simulink model "new3"  (R2025a)
settings: Solver=VariableStepAuto  StartTime=0.0  StopTime=2  RelTol=1e-3
undefined symbols (not defined in the file): g, Rs, Rsl, Rw, Ry
libraries: fl_lib x40, nesl_utility x14, ee_lib x12, slpidlib x3, spsFirstOrderFilterLib x1, spsOnDelayLib x1, simulink x1, spsabctodq0Lib x1
settings Model: SimulationMode=accelerator  Creator=maska  LastModifiedBy=maska

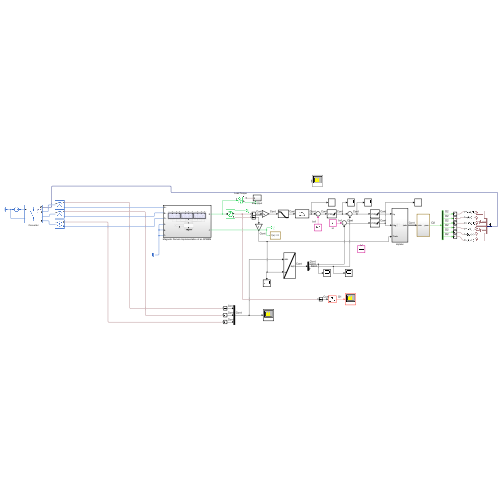
[thumbnail: Simulink's stored preview of the top-level diagram]
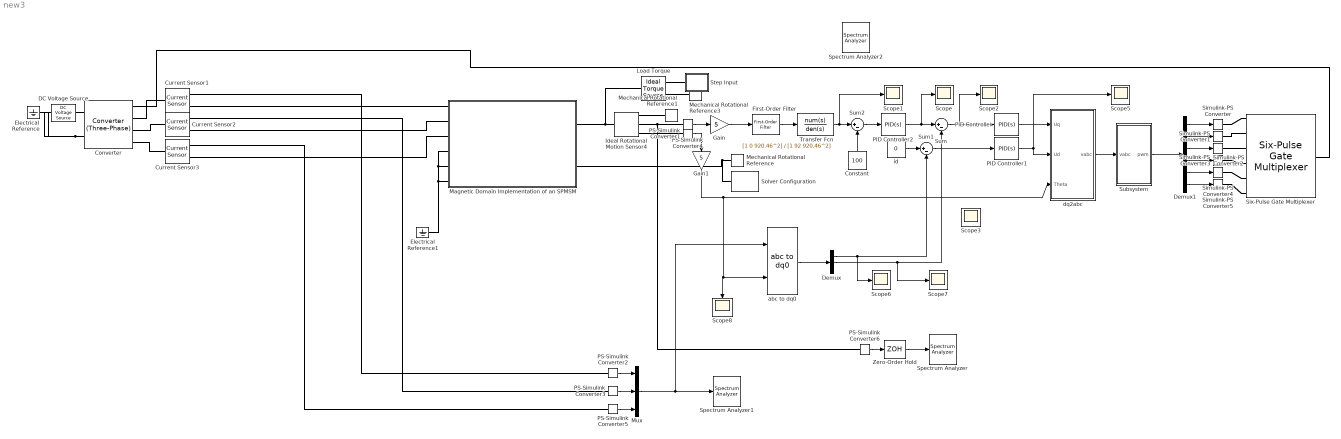
== system new3 ==
  Constant : Constant  Value=100
  Converter : ee_lib/Semiconductors & Converters/Converters/Converter (Three-Phase)  port_option=ee.enum.threePhasePort.expanded  fidelity_option=ee.enum.converters.fidelity.detailed  device_type=3  showThermalPort=false  K=0  Vth=0.5 V  Vgt=1 V  Vgt_off=-1 V  Ih=1 A  Vf=0.8 V  Ron=0.001 Ohm  Rds=0.001 Ohm  Goff=1e-5 1/Ohm  Eon_scalar=22.86e-3 J  Eoff_scalar=17.14e-3 J  Eoff_natural_commutation=10e-3 J  Voff=300 V  Iout_scalar=600 A  onCurrentMeasDelay=0 s  useCurrentFromPreviousCycle=false  useVoltageFromPreviousCycle=false  diode_param=2  diode_Vf=0.8 V  diode_Ron=0.001 Ohm  diode_Goff=1e-5 1/Ohm  diode_C=50 nF  diode_iRM=-235 A  diode_iF=300 A  diode_idot=-50 A/us  diode_trr_param=1  diode_trr_factor=3  diode_trr=15 us  diode_Qrr=1.5e+3 s*uA  diode_rec_loss_model=ee.enum.diode.reverseRecoveryModel.fixed  diode_ErecVal=0 J  diode_scaleWithIandV=false  diode_ErecMat=zeros(2, 3) J  diode_TjrecVec=[298.15, 398.15] K  diode_IfrecVec=[.1, 1, 10] A  diode_IrecVal=10 A  diode_VrecVal=10 V  diode_tFilter=1 / 1000 / 100 s  thermal_network_parameterization=ee.enum.thermalNetworkTopology.external  Rth=[.08, .5] K/W  Rth_Cauer=[.08, .1, .5] K/W  Rth_Foster=[.08, .14, .22, .16] K/W  thermal_mass_parameterization=ee.enum.thermalNetwork.timeconstant  thermal_mass=[.01, .5] J/K  thermal_mass_Cauer=[.01, .1, .5] J/K  thermal_mass_Foster=[.001, .005, .05, .5] J/K  thermal_time_constant=[.001, .2] s  thermal_time_constant_Cauer=[.001, .1, .2] s  thermal_time_constant_Foster=[7e-05, .0007, .01, .08] s  thermal_mass_initial_temperatures=[25, 25] degC  thermal_mass_initial_temperatures_Cauer=[25, 25, 25] degC  junction_thermal_mass=0.01 J/K  Tvec_initial_Foster=[25, 25, 25, 25] degC  snubber_type=0  Cs=1e-7 F  Rs=0.1 Ohm  Vce_loss=[0, 150, 300] V
      settings: InternalSimscapePortConfiguration="{\"Bottom\":[],\"Left\":[{\"id\":\"G\",\"label\":\"G\",\"type\":\"foundation.electrical.twelve_phase\"},{\"id\":\"a\",\"label\":\"a\",\"type\":\"foundation.electrical.electrical\"},{\"id\":\"b\",\"label\":\"b\",\"type\":\"foundation.electrical.electrical\"},{\"id\":\"c\",\"label\":\"c\",\"type\":\"foundation.electrical.electrical\"}],\"Right\":[{\"id\":\"p\",\"label\":\"+\",\"type\":\"foundation.electrical.electrical\"},{\"id\":\"n\",\"label\":\"-\",\"type\":\"foundation.electrical.electrical\"}],\"Top\":[]}"
  Current Sensor1 : fl_lib/Electrical/Electrical Sensors/Current Sensor
  Current Sensor2 : fl_lib/Electrical/Electrical Sensors/Current Sensor
  Current Sensor3 : fl_lib/Electrical/Electrical Sensors/Current Sensor
  DC Voltage Source : fl_lib/Electrical/Electrical Sources/DC Voltage Source  v0=750 V
  Demux : Demux  Outputs=3
  Demux1 : Demux  Outputs=6
  Electrical Reference : fl_lib/Electrical/Electrical Elements/Electrical Reference
  Electrical Reference1 : fl_lib/Electrical/Electrical Elements/Electrical Reference
  First-Order Filter : spsFirstOrderFilterLib/First-Order Filter  FilterType=Lowpass  Tc=0.04  Ts=0  Initialize=on  Vac_Init=[0, 0, 60]  Vdc_Init=0  PlotResponse=off  FreqRange="[0,  200,  1]"
  Gain : Gain  Gain=5
  Gain1 : Gain  Gain=5
  Ideal Rotational Motion Sensor4 : fl_lib/Mechanical/Mechanical Sensors/Ideal Rotational Motion Sensor  reference=foundation.enum.MeasurementReference.difference  acceleration_port=false  velocity_port=true  position_port=true  wrap_angle=false  offset=0 rad
  Load Torque : fl_lib/Mechanical/Mechanical Sources/Ideal Torque Source
  Magnetic Domain Implementation of an SPMSM : Subsystem
  Mechanical Rotational Reference : fl_lib/Mechanical/Rotational Elements/Mechanical Rotational Reference
  Mechanical Rotational Reference1 : fl_lib/Mechanical/Rotational Elements/Mechanical Rotational Reference
  Mechanical Rotational Reference3 : fl_lib/Mechanical/Rotational Elements/Mechanical Rotational Reference
  Mux : Mux  Inputs=3
  PID Controller : slpidlib/PID Controller  Controller=PID  Form=Parallel  TimeDomain=Continuous-time  UseExternalTs=off  SampleTime=-1  IntegratorMethod=Forward Euler  FilterMethod=Forward Euler  ControllerParametersSource=internal  P=1.95  I=0.85  UseKiTs=off  D=0  UseExternalDerivativeSource=off  N=100  UseFilter=on  TunerSelectOption=Transfer Function Based (PID Tuner App)  InitialConditionSource=internal  InitialConditionForIntegrator=0  InitialConditionForFilter=0  DifferentiatorICPrevScaledInput=0  ExternalReset=none  TrackingMode=off  Kt=1  LimitOutput=on  SatLimitsSource=internal  UpperSaturationLimit=1000  LowerSaturationLimit=-1000  LinearizeAsGain=on  AntiWindupMode=none  Kb=1  LimitIntegrator=on  UpperIntegratorSaturationLimit=100  LowerIntegratorSaturationLimit=-100  POutMin=[]  POutMax=[]  IOutMin=[]  IOutMax=[]  DOutMin=[]  DOutMax=[]  NOutMin=[]  NOutMax=[]  SumOutMin=[]  SumOutMax=[]  SaturationOutMin=[]  SaturationOutMax=[]  PParamMin=[]  PParamMax=[]  IParamMin=[]  IParamMax=[]  DParamMin=[]  DParamMax=[]  NParamMin=[]  NParamMax=[]  KbParamMin=[]  KbParamMax=[]  KtParamMin=[]  KtParamMax=[]  KbOutMin=[]  KbOutMax=[]  KtOutMin=[]  KtOutMax=[]  IntegratorOutMin=[]  IntegratorOutMax=[]  FilterOutMin=[]  FilterOutMax=[]  SumI1OutMin=[]  SumI1OutMax=[]  SumI2OutMin=[]  SumI2OutMax=[]  SumI3OutMin=[]  SumI3OutMax=[]  SumI4OutMin=[]  SumI4OutMax=[]  SumDOutMin=[]  SumDOutMax=[]  DifferentiatorOutMin=[]  DifferentiatorOutMax=[]  FilterDiffOutCoefMin=[]  FilterDiffOutCoefMax=[]  ReciprocalOutMin=[]  ReciprocalOutMax=[]  SumDenOutMin=[]  SumDenOutMax=[]  SumNumOutMin=[]  SumNumOutMax=[]  DivideOutMin=[]  DivideOutMax=[]  UdiffTsProdOutMin=[]  UdiffTsProdOutMax=[]  NTsProdOutMin=[]  NTsProdOutMax=[]  UintegralTsProdOutMin=[]  UintegralTsProdOutMax=[]  UngainTsProdOutMin=[]  UngainTsProdOutMax=[]  ClampingZeroOutDataTypeStr=Inherit: Inherit via back propagation  ClampingZeroOutMin=[]  ClampingZeroOutMax=[]  FilterDenConstantOutDataTypeStr=Inherit: Inherit via back propagation  FilterDenConstantOutMin=[]  FilterDenConstantOutMax=[]  PCopyOutDataTypeStr=Inherit: Inherit via back propagation  PCopyOutMin=[]  PCopyOutMax=[]  NCopyOutDataTypeStr=Inherit: Inherit via back propagation  NCopyOutMin=[]  NCopyOutMax=[]  IntegratorContinuousStateAttributes=''  IntegratorStateMustResolveToSignalObject=off  IntegratorRTWStateStorageClass=Auto  FilterContinuousStateAttributes=''  FilterStateMustResolveToSignalObject=off  FilterRTWStateStorageClass=Auto  ParallelPVariant=InternalParameters  IdealPVariant=Disabled  IVariant=InternalParameters  DVariant=InternalParameters  IntegratorVariant=Continuous  SatVariant=Enabled  AWVariant=Passthrough  PCopyVariant=Disabled  TRVariant=Disabled  FdbkBlocksVariant=Forward  IdealPFdbkVariant=Disabled  SatFdbkVariant=Disabled  DerivativeFilterVariant=ContFilter  NVariant=InternalParameters  NCopyVariant=Disabled  FilterICVariant=InternalICsFilter  IntegratorICVariant=InternalICs  ExternalResetVariant=Disabled  TRSumVariant=Passthrough  SumFdbkVariant=Disabled  SumVariant=Sum_PID  TsampFilterVariant=InternalTs  TsampNgainVariant=Passthrough  TsampIntegralVariant=Disabled_SignalSpec  ExternalSaturationOutDataTypeStr=Inherit: Same as second input  DerivativeSourceVariant=ErrorSignal  PreIntVariant=InternalPreInt
  PID Controller1 : slpidlib/PID Controller  Controller=PID  Form=Parallel  TimeDomain=Continuous-time  UseExternalTs=off  SampleTime=-1  IntegratorMethod=Forward Euler  FilterMethod=Forward Euler  ControllerParametersSource=internal  P=1.95  I=0.85  UseKiTs=off  D=0  UseExternalDerivativeSource=off  N=100  UseFilter=on  TunerSelectOption=Transfer Function Based (PID Tuner App)  InitialConditionSource=internal  InitialConditionForIntegrator=0  InitialConditionForFilter=0  DifferentiatorICPrevScaledInput=0  ExternalReset=none  TrackingMode=off  Kt=1  LimitOutput=on  SatLimitsSource=internal  UpperSaturationLimit=1000  LowerSaturationLimit=-1000  LinearizeAsGain=on  AntiWindupMode=none  Kb=1  LimitIntegrator=on  UpperIntegratorSaturationLimit=100  LowerIntegratorSaturationLimit=-100  POutMin=[]  POutMax=[]  IOutMin=[]  IOutMax=[]  DOutMin=[]  DOutMax=[]  NOutMin=[]  NOutMax=[]  SumOutMin=[]  SumOutMax=[]  SaturationOutMin=[]  SaturationOutMax=[]  PParamMin=[]  PParamMax=[]  IParamMin=[]  IParamMax=[]  DParamMin=[]  DParamMax=[]  NParamMin=[]  NParamMax=[]  KbParamMin=[]  KbParamMax=[]  KtParamMin=[]  KtParamMax=[]  KbOutMin=[]  KbOutMax=[]  KtOutMin=[]  KtOutMax=[]  IntegratorOutMin=[]  IntegratorOutMax=[]  FilterOutMin=[]  FilterOutMax=[]  SumI1OutMin=[]  SumI1OutMax=[]  SumI2OutMin=[]  SumI2OutMax=[]  SumI3OutMin=[]  SumI3OutMax=[]  SumI4OutMin=[]  SumI4OutMax=[]  SumDOutMin=[]  SumDOutMax=[]  DifferentiatorOutMin=[]  DifferentiatorOutMax=[]  FilterDiffOutCoefMin=[]  FilterDiffOutCoefMax=[]  ReciprocalOutMin=[]  ReciprocalOutMax=[]  SumDenOutMin=[]  SumDenOutMax=[]  SumNumOutMin=[]  SumNumOutMax=[]  DivideOutMin=[]  DivideOutMax=[]  UdiffTsProdOutMin=[]  UdiffTsProdOutMax=[]  NTsProdOutMin=[]  NTsProdOutMax=[]  UintegralTsProdOutMin=[]  UintegralTsProdOutMax=[]  UngainTsProdOutMin=[]  UngainTsProdOutMax=[]  ClampingZeroOutDataTypeStr=Inherit: Inherit via back propagation  ClampingZeroOutMin=[]  ClampingZeroOutMax=[]  FilterDenConstantOutDataTypeStr=Inherit: Inherit via back propagation  FilterDenConstantOutMin=[]  FilterDenConstantOutMax=[]  PCopyOutDataTypeStr=Inherit: Inherit via back propagation  PCopyOutMin=[]  PCopyOutMax=[]  NCopyOutDataTypeStr=Inherit: Inherit via back propagation  NCopyOutMin=[]  NCopyOutMax=[]  IntegratorContinuousStateAttributes=''  IntegratorStateMustResolveToSignalObject=off  IntegratorRTWStateStorageClass=Auto  FilterContinuousStateAttributes=''  FilterStateMustResolveToSignalObject=off  FilterRTWStateStorageClass=Auto  ParallelPVariant=InternalParameters  IdealPVariant=Disabled  IVariant=InternalParameters  DVariant=InternalParameters  IntegratorVariant=Continuous  SatVariant=Enabled  AWVariant=Passthrough  PCopyVariant=Disabled  TRVariant=Disabled  FdbkBlocksVariant=Forward  IdealPFdbkVariant=Disabled  SatFdbkVariant=Disabled  DerivativeFilterVariant=ContFilter  NVariant=InternalParameters  NCopyVariant=Disabled  FilterICVariant=InternalICsFilter  IntegratorICVariant=InternalICs  ExternalResetVariant=Disabled  TRSumVariant=Passthrough  SumFdbkVariant=Disabled  SumVariant=Sum_PID  TsampFilterVariant=InternalTs  TsampNgainVariant=Passthrough  TsampIntegralVariant=Disabled_SignalSpec  ExternalSaturationOutDataTypeStr=Inherit: Same as second input  DerivativeSourceVariant=ErrorSignal  PreIntVariant=InternalPreInt
  PID Controller2 : slpidlib/PID Controller  Controller=PID  Form=Parallel  TimeDomain=Continuous-time  UseExternalTs=off  SampleTime=-1  IntegratorMethod=Forward Euler  FilterMethod=Forward Euler  ControllerParametersSource=internal  P=0.008  I=0.00007  UseKiTs=off  D=0  UseExternalDerivativeSource=off  N=100  UseFilter=on  TunerSelectOption=Transfer Function Based (PID Tuner App)  InitialConditionSource=internal  InitialConditionForIntegrator=0  InitialConditionForFilter=0  DifferentiatorICPrevScaledInput=0  ExternalReset=none  TrackingMode=off  Kt=1  LimitOutput=on  SatLimitsSource=internal  UpperSaturationLimit=100  LowerSaturationLimit=-100  LinearizeAsGain=on  AntiWindupMode=none  Kb=1  LimitIntegrator=on  UpperIntegratorSaturationLimit=100  LowerIntegratorSaturationLimit=-100  POutMin=[]  POutMax=[]  IOutMin=[]  IOutMax=[]  DOutMin=[]  DOutMax=[]  NOutMin=[]  NOutMax=[]  SumOutMin=[]  SumOutMax=[]  SaturationOutMin=[]  SaturationOutMax=[]  PParamMin=[]  PParamMax=[]  IParamMin=[]  IParamMax=[]  DParamMin=[]  DParamMax=[]  NParamMin=[]  NParamMax=[]  KbParamMin=[]  KbParamMax=[]  KtParamMin=[]  KtParamMax=[]  KbOutMin=[]  KbOutMax=[]  KtOutMin=[]  KtOutMax=[]  IntegratorOutMin=[]  IntegratorOutMax=[]  FilterOutMin=[]  FilterOutMax=[]  SumI1OutMin=[]  SumI1OutMax=[]  SumI2OutMin=[]  SumI2OutMax=[]  SumI3OutMin=[]  SumI3OutMax=[]  SumI4OutMin=[]  SumI4OutMax=[]  SumDOutMin=[]  SumDOutMax=[]  DifferentiatorOutMin=[]  DifferentiatorOutMax=[]  FilterDiffOutCoefMin=[]  FilterDiffOutCoefMax=[]  ReciprocalOutMin=[]  ReciprocalOutMax=[]  SumDenOutMin=[]  SumDenOutMax=[]  SumNumOutMin=[]  SumNumOutMax=[]  DivideOutMin=[]  DivideOutMax=[]  UdiffTsProdOutMin=[]  UdiffTsProdOutMax=[]  NTsProdOutMin=[]  NTsProdOutMax=[]  UintegralTsProdOutMin=[]  UintegralTsProdOutMax=[]  UngainTsProdOutMin=[]  UngainTsProdOutMax=[]  ClampingZeroOutDataTypeStr=Inherit: Inherit via back propagation  ClampingZeroOutMin=[]  ClampingZeroOutMax=[]  FilterDenConstantOutDataTypeStr=Inherit: Inherit via back propagation  FilterDenConstantOutMin=[]  FilterDenConstantOutMax=[]  PCopyOutDataTypeStr=Inherit: Inherit via back propagation  PCopyOutMin=[]  PCopyOutMax=[]  NCopyOutDataTypeStr=Inherit: Inherit via back propagation  NCopyOutMin=[]  NCopyOutMax=[]  IntegratorContinuousStateAttributes=''  IntegratorStateMustResolveToSignalObject=off  IntegratorRTWStateStorageClass=Auto  FilterContinuousStateAttributes=''  FilterStateMustResolveToSignalObject=off  FilterRTWStateStorageClass=Auto  ParallelPVariant=InternalParameters  IdealPVariant=Disabled  IVariant=InternalParameters  DVariant=InternalParameters  IntegratorVariant=Continuous  SatVariant=Enabled  AWVariant=Passthrough  PCopyVariant=Disabled  TRVariant=Disabled  FdbkBlocksVariant=Forward  IdealPFdbkVariant=Disabled  SatFdbkVariant=Disabled  DerivativeFilterVariant=ContFilter  NVariant=InternalParameters  NCopyVariant=Disabled  FilterICVariant=InternalICsFilter  IntegratorICVariant=InternalICs  ExternalResetVariant=Disabled  TRSumVariant=Passthrough  SumFdbkVariant=Disabled  SumVariant=Sum_PID  TsampFilterVariant=InternalTs  TsampNgainVariant=Passthrough  TsampIntegralVariant=Disabled_SignalSpec  ExternalSaturationOutDataTypeStr=Inherit: Same as second input  DerivativeSourceVariant=ErrorSignal  PreIntVariant=InternalPreInt
  PS-Simulink Converter{1..6} (6 alike) : nesl_utility/PS-Simulink Converter  PhysicalDomain=network_engine_domain  SubClassName=ps_output  LeftPortType=input  RightPortType=output  PseudoPeriodic=off  Frequencies=[]  VectorFormat=inherit  Unit=inherit  AffineConversion=off
  Scope{,1..3,5..8} (8 alike) : Scope
      Scope settings: ActiveDisplayYMinimum=-4.019417563087452  ActiveDisplayYMaximum=1.1746832168582009
      Scope1 settings: ActiveDisplayYMinimum=-11.267228325018072  ActiveDisplayYMaximum=101.40505492516266
      Scope2 settings: ActiveDisplayYMinimum=-27.834658782595159  ActiveDisplayYMaximum=26.640626012143759  DataLoggingVariableName=ScopeData2
      Scope3 settings: ActiveDisplayYMinimum=-20.005283078213854  ActiveDisplayYMaximum=19.374157195669472  DataLoggingVariableName=ScopeData3
      Scope5 settings: ActiveDisplayYMinimum=-53.508802129582079  ActiveDisplayYMaximum=53.186558135240951  DataLoggingVariableName=ScopeData5
      Scope6 settings: ActiveDisplayYMinimum=-1437.9474938047751  ActiveDisplayYMaximum=1776.8392107438344  DataLoggingVariableName=ScopeData6
      Scope7 settings: ActiveDisplayYMinimum=-2.8426588150958878  ActiveDisplayYMaximum=1.0409285736394622  DataLoggingVariableName=ScopeData7
      Scope8 settings: ActiveDisplayYMinimum=10.636225564991161  ActiveDisplayYMaximum=10.664194284729955  DataLoggingVariableName=ScopeData8
  Simulink-PS Converter{,1..5} (6 alike) : nesl_utility/Simulink-PS Converter  PhysicalDomain=network_engine_domain  SubClassName=ps_input  LeftPortType=input  RightPortType=output  PseudoPeriodic=off  Frequencies=[]  NoiseDistribution=none  NoiseParameters=[]  Unit=1  AffineConversion=off  FilteringAndDerivatives=provide  SimscapeFilterOrder=1  InputFilterTimeConstant=0.001  UdotUserProvided=0
  Six-Pulse Gate Multiplexer : ee_lib/Semiconductors & Converters/Converters/Six-Pulse Gate Multiplexer  port_option=ee.enum.controlport.ps
  Solver Configuration : nesl_utility/Solver Configuration  PhysicalDomain=network_engine_domain  SubClassName=solver  LeftPortType=input  RightPortType=generic  Tones=[]  Harmonics=[]  SimulateNoise=off  Profile=off  UseLocalSampling=off  EnableSwitchedLinearOptims=on  FrequencyDomain=off  UseCCode=off  RelTol=0.001  AbsTol=1e-06  MinStep=1e-09  ToWorkspace=off  RevertToSquareIcSolve=off  NumHomotopyIterations=100  PhasorMode=off  PhasorModeNumHarmonics=1  ConsistencySolver=NEWTON_FTOL  IndexReductionMethod=DerivativeReplacement  DoDC=off  ResidualTolerance=1e-09  ConsistencyTolSource=GLOBAL  ConsistencyAbsTol=0.001  ConsistencyRelTol=0.001  ConsistencyTolFactor=0.001  UseLocalSolver=off  LocalSolverChoice=NE_BACKWARD_EULER_ADVANCER  ResolveIndetEquations=on  FunctionEvalNumThread=1  LocalSolverSampleTime=0.0001  DoFixedCost=off  MaxNonlinIter=3  MaxModeIter=2  ComputeImpulses=off  ImpulseIterations=1  LinearAlgebra=auto  LinearAlgebraNumThread=0  EquationFormulation=NE_TIME_EF  DelaysMemoryBudget=1024  AutomaticFiltering=on  FilteringTimeConstant=0.001  PartitionStorageMethod=AS_NEEDED  PartitionMemoryBudget=1024  PartitionMethod=ROBUST  MultibodyUseLocalSolver=off  MultibodyLocalSolverChoice=ODE1  MultibodyLocalSolverSampleTime=0.001
  Spectrum Analyzer : SpectrumAnalyzer  WindowPosition=[231.000000,114.000000,800.000000,483.000000,]  ScopeFrameLocation=window  SampleRate=44.1e3  PlotAsTwoSidedSpectrum=off  FrequencyScale=Log  WindowInvariantSamplesPerUpdate=on  FrequencySpan=Start and stop frequencies  StartFrequency=0  StopFrequency=50000  MaximizeAxes=Off  YLimits=[-34.3366 63.0554]  SelectedToolstripTab=spectrumAnalyzerToolstrip.measurementsTab
  Spectrum Analyzer1 : SpectrumAnalyzer  WindowPosition=[37.000000,290.000000,800.000000,483.000000,]  ScopeFrameLocation=window  SampleRate=44.1e3  PlotAsTwoSidedSpectrum=off  FrequencyScale=Log  WindowInvariantSamplesPerUpdate=on  FrequencySpan=Start and stop frequencies  StartFrequency=0  StopFrequency=50000  MaximizeAxes=Off  YLimits=[-64.8278 131.059]  SelectedToolstripTab=spectrumAnalyzerToolstrip.measurementsTab
  Spectrum Analyzer2 : SpectrumAnalyzer  WindowPosition=[959.000000,121.000000,800.000000,483.000000,]  ScopeFrameLocation=window  SampleRate=44.1e3  PlotAsTwoSidedSpectrum=off  FrequencyScale=Log  WindowInvariantSamplesPerUpdate=on  FrequencySpan=Start and stop frequencies  StartFrequency=0  StopFrequency=50000  MaximizeAxes=Off  YLimits=[-3603.4449 -2802.6794]  SelectedToolstripTab=spectrumAnalyzerToolstrip.measurementsTab
  Step Input : Subsystem
  Subsystem : Subsystem
  Sum : Sum  Inputs=|+-
  Sum1 : Sum  Inputs=|+-
  Sum2 : Sum  Inputs=|+-
  Transfer Fcn : TransferFcn  Numerator=[1 0 920.46^2]  Denominator=[1 92 920.46^2]
  Zero-Order Hold : ZeroOrderHold  SampleTime=1e-6
  abc to dq0 : spsabctodq0Lib/abc to dq0  Alignment=90 degrees behind phase A axis
  dq2abc : Subsystem
  id : Constant  Value=0
  wires:
  Mux/1 -> abc to dq0/1, Spectrum Analyzer1/1
  Demux1/5 -> Simulink-PS Converter4/1
  Demux1/4 -> Simulink-PS Converter3/1
  PS-Simulink Converter5/1 -> Mux/3
  PS-Simulink Converter2/1 -> Mux/1
  Demux/1 -> Sum1/2, Scope6/1
  Demux/2 -> Scope7/1, Sum/2
  Demux1/3 -> Simulink-PS Converter2/1
  PS-Simulink Converter6/1 -> Zero-Order Hold/1
  PS-Simulink Converter1/1 -> Gain1/1
  id/1 -> Sum1/1
  Constant/1 -> Sum2/2
  Gain1/1 -> abc to dq0/2, Scope8/1, dq2abc/3(Theta)
  dq2abc/1(vabc) -> Subsystem/1(vabc)
  abc to dq0/1 -> Demux/1
  Demux1/2 -> Simulink-PS Converter1/1
  Zero-Order Hold/1 -> Spectrum Analyzer/1
  Demux1/1 -> Simulink-PS Converter/1
  Demux1/6 -> Simulink-PS Converter5/1
  PS-Simulink Converter3/1 -> Mux/2
  PID Controller1/1 -> dq2abc/2(Ud), Scope5/1
  Subsystem/1(pwm) -> Demux1/1
  Sum2/1 -> PID Controller2/1
  PID Controller2/1 -> Scope/1, Sum/1
  PID Controller/1 -> dq2abc/1(Uq)
  PS-Simulink Converter4/1 -> Gain/1
  Gain/1 -> First-Order Filter/1
  First-Order Filter/1 -> Transfer Fcn/1
  Sum/1 -> PID Controller/1, Scope2/1
  Sum1/1 -> PID Controller1/1
  Transfer Fcn/1 -> Scope1/1, Sum2/1
  connections:
  Mechanical Rotational Reference/LConn1 -- Magnetic Domain Implementation of an SPMSM/RConn2 -- Solver Configuration/RConn1
  Converter/RConn2 -- DC Voltage Source/RConn1 -- Electrical Reference/LConn1
  Simulink-PS Converter1/RConn1 -- Six-Pulse Gate Multiplexer/LConn2
  PS-Simulink Converter3/LConn1 -- Current Sensor2/RConn1
  Ideal Rotational Motion Sensor4/LConn1 -- Load Torque/LConn1 -- Magnetic Domain Implementation of an SPMSM/RConn1
  Converter/LConn4 -- Current Sensor3/LConn1
  PS-Simulink Converter2/LConn1 -- Current Sensor1/RConn1
  Simulink-PS Converter5/RConn1 -- Six-Pulse Gate Multiplexer/LConn6
  Converter/LConn1 -- Six-Pulse Gate Multiplexer/RConn1
  Simulink-PS Converter2/RConn1 -- Six-Pulse Gate Multiplexer/LConn3
  DC Voltage Source/LConn1 -- Converter/RConn1
  PS-Simulink Converter5/LConn1 -- Current Sensor3/RConn1
  Simulink-PS Converter3/RConn1 -- Six-Pulse Gate Multiplexer/LConn4
  Electrical Reference1/LConn1 -- Magnetic Domain Implementation of an SPMSM/LConn4 -- Magnetic Domain Implementation of an SPMSM/LConn5 -- Magnetic Domain Implementation of an SPMSM/LConn6
  Simulink-PS Converter4/RConn1 -- Six-Pulse Gate Multiplexer/LConn5
  Simulink-PS Converter/RConn1 -- Six-Pulse Gate Multiplexer/LConn1
  Converter/LConn3 -- Current Sensor2/LConn1
  Converter/LConn2 -- Current Sensor1/LConn1
  Magnetic Domain Implementation of an SPMSM/LConn1 -- Current Sensor1/RConn2
  Magnetic Domain Implementation of an SPMSM/LConn2 -- Current Sensor2/RConn2
  Magnetic Domain Implementation of an SPMSM/LConn3 -- Current Sensor3/RConn2
  Mechanical Rotational Reference3/LConn1 -- Load Torque/RConn2
  Step Input/LConn1 -- Load Torque/RConn1
  Ideal Rotational Motion Sensor4/RConn1 -- Mechanical Rotational Reference1/LConn1
  Ideal Rotational Motion Sensor4/RConn3 -- PS-Simulink Converter1/LConn1
  Ideal Rotational Motion Sensor4/RConn2 -- PS-Simulink Converter6/LConn1 -- PS-Simulink Converter4/LConn1

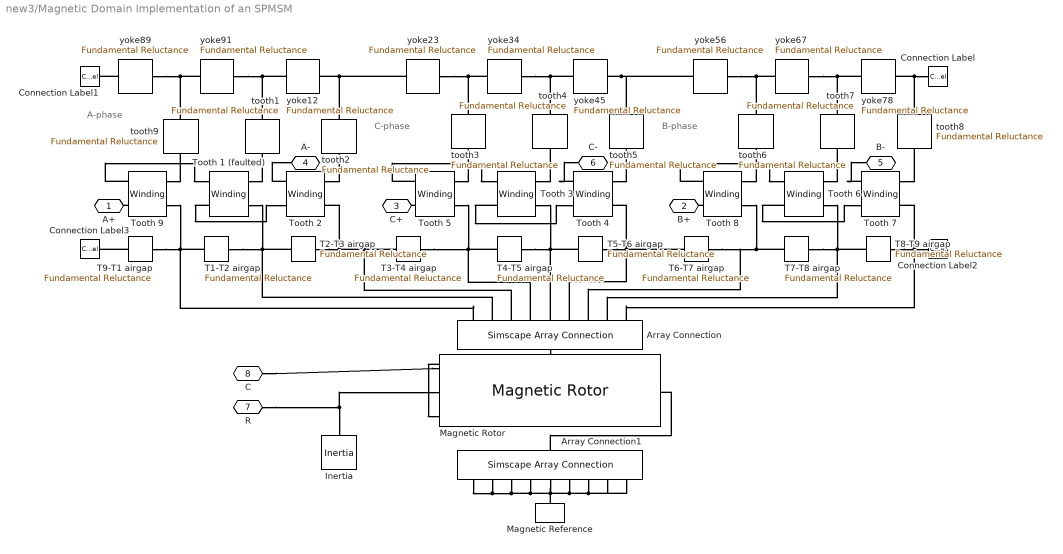
== system new3/Magnetic Domain Implementation of an SPMSM ==
  note: A-phase
  note: C-phase
  note: B-phase
  Array Connection : SimscapeArrayConnection  Domain=foundation.magnetic.magnetic  NumScalarElements=9
  Array Connection1 : SimscapeArrayConnection  Domain=foundation.magnetic.magnetic  NumScalarElements=9
  Connection Label : ConnectionLabel  Label=Y
  Connection Label1 : ConnectionLabel  Label=Y
  Connection Label2 : ConnectionLabel  Label=SL
  Connection Label3 : ConnectionLabel  Label=SL
  Inertia : fl_lib/Mechanical/Rotational Elements/Inertia  inertia=J kg*m^2  num_ports=foundation.enum.numPorts2.one  w_specify=on  w_priority=None  w=0 rad/s  w_nominal_specify=off  w_nominal_value=1  w_nominal_unit=rad/s  t_specify=off  t_priority=High  t=0 N*m  t_nominal_specify=off  t_nominal_value=1  t_nominal_unit=N*m
  Magnetic Reference : fl_lib/Magnetic/Magnetic Elements/Magnetic Reference
      settings: InternalSimscapePortConfiguration="{\"Bottom\":[],\"Left\":[{\"id\":\"M\",\"label\":\"\",\"type\":\"foundation.magnetic.magnetic\"}],\"Right\":[],\"Top\":[]}"
  Magnetic Rotor : ee_lib/Electromechanical/Magnetic Rotor  Nr=5  Ns=Ns  B0=B0 T  lm=lm mm  mur=1.05  g=g mm  r=r mm  l=l mm
      settings: InternalSimscapePortConfiguration="{\"Bottom\":[{\"id\":\"S\",\"label\":\"S\",\"type\":\"foundation.magnetic.magnetic\"}],\"Left\":[{\"id\":\"C\",\"label\":\"C\",\"type\":\"foundation.mechanical.rotational.rotational\"},{\"id\":\"R\",\"label\":\"R\",\"type\":\"foundation.mechanical.rotational.rotational\"}],\"Right\":[],\"Top\":[{\"id\":\"N\",\"label\":\"N\",\"type\":\"foundation.magnetic.magnetic\"}]}"
  T1-T2 airgap : fl_lib/Magnetic/Magnetic Elements/Fundamental Reluctance  R=Rsl 1/H  phi_specify=off  phi_priority=None  phi=0 Wb  phi_nominal_specify=off  phi_nominal_value=1  phi_nominal_unit=Wb  mmf_specify=off  mmf_priority=None  mmf=0 A  mmf_nominal_specify=off  mmf_nominal_value=1  mmf_nominal_unit=A
      settings: InternalSimscapePortConfiguration="{\"Bottom\":[],\"Left\":[{\"id\":\"N\",\"label\":\"N\",\"type\":\"foundation.magnetic.magnetic\"}],\"Right\":[{\"id\":\"S\",\"label\":\"S\",\"type\":\"foundation.magnetic.magnetic\"}],\"Top\":[]}"
  T2-T3 airgap : fl_lib/Magnetic/Magnetic Elements/Fundamental Reluctance  R=Rsl 1/H  phi_specify=off  phi_priority=None  phi=0 Wb  phi_nominal_specify=off  phi_nominal_value=1  phi_nominal_unit=Wb  mmf_specify=off  mmf_priority=None  mmf=0 A  mmf_nominal_specify=off  mmf_nominal_value=1  mmf_nominal_unit=A
      settings: InternalSimscapePortConfiguration="{\"Bottom\":[],\"Left\":[{\"id\":\"N\",\"label\":\"N\",\"type\":\"foundation.magnetic.magnetic\"}],\"Right\":[{\"id\":\"S\",\"label\":\"S\",\"type\":\"foundation.magnetic.magnetic\"}],\"Top\":[]}"
  T3-T4 airgap : fl_lib/Magnetic/Magnetic Elements/Fundamental Reluctance  R=Rsl 1/H  phi_specify=off  phi_priority=None  phi=0 Wb  phi_nominal_specify=off  phi_nominal_value=1  phi_nominal_unit=Wb  mmf_specify=off  mmf_priority=None  mmf=0 A  mmf_nominal_specify=off  mmf_nominal_value=1  mmf_nominal_unit=A
      settings: InternalSimscapePortConfiguration="{\"Bottom\":[],\"Left\":[{\"id\":\"N\",\"label\":\"N\",\"type\":\"foundation.magnetic.magnetic\"}],\"Right\":[{\"id\":\"S\",\"label\":\"S\",\"type\":\"foundation.magnetic.magnetic\"}],\"Top\":[]}"
  T4-T5 airgap : fl_lib/Magnetic/Magnetic Elements/Fundamental Reluctance  R=Rsl 1/H  phi_specify=off  phi_priority=None  phi=0 Wb  phi_nominal_specify=off  phi_nominal_value=1  phi_nominal_unit=Wb  mmf_specify=off  mmf_priority=None  mmf=0 A  mmf_nominal_specify=off  mmf_nominal_value=1  mmf_nominal_unit=A
      settings: InternalSimscapePortConfiguration="{\"Bottom\":[],\"Left\":[{\"id\":\"N\",\"label\":\"N\",\"type\":\"foundation.magnetic.magnetic\"}],\"Right\":[{\"id\":\"S\",\"label\":\"S\",\"type\":\"foundation.magnetic.magnetic\"}],\"Top\":[]}"
  T5-T6 airgap : fl_lib/Magnetic/Magnetic Elements/Fundamental Reluctance  R=Rsl 1/H  phi_specify=off  phi_priority=None  phi=0 Wb  phi_nominal_specify=off  phi_nominal_value=1  phi_nominal_unit=Wb  mmf_specify=off  mmf_priority=None  mmf=0 A  mmf_nominal_specify=off  mmf_nominal_value=1  mmf_nominal_unit=A
      settings: InternalSimscapePortConfiguration="{\"Bottom\":[],\"Left\":[{\"id\":\"N\",\"label\":\"N\",\"type\":\"foundation.magnetic.magnetic\"}],\"Right\":[{\"id\":\"S\",\"label\":\"S\",\"type\":\"foundation.magnetic.magnetic\"}],\"Top\":[]}"
  T6-T7 airgap : fl_lib/Magnetic/Magnetic Elements/Fundamental Reluctance  R=Rsl 1/H  phi_specify=off  phi_priority=None  phi=0 Wb  phi_nominal_specify=off  phi_nominal_value=1  phi_nominal_unit=Wb  mmf_specify=off  mmf_priority=None  mmf=0 A  mmf_nominal_specify=off  mmf_nominal_value=1  mmf_nominal_unit=A
      settings: InternalSimscapePortConfiguration="{\"Bottom\":[],\"Left\":[{\"id\":\"N\",\"label\":\"N\",\"type\":\"foundation.magnetic.magnetic\"}],\"Right\":[{\"id\":\"S\",\"label\":\"S\",\"type\":\"foundation.magnetic.magnetic\"}],\"Top\":[]}"
  T7-T8 airgap : fl_lib/Magnetic/Magnetic Elements/Fundamental Reluctance  R=Rsl 1/H  phi_specify=off  phi_priority=None  phi=0 Wb  phi_nominal_specify=off  phi_nominal_value=1  phi_nominal_unit=Wb  mmf_specify=off  mmf_priority=None  mmf=0 A  mmf_nominal_specify=off  mmf_nominal_value=1  mmf_nominal_unit=A
      settings: InternalSimscapePortConfiguration="{\"Bottom\":[],\"Left\":[{\"id\":\"N\",\"label\":\"N\",\"type\":\"foundation.magnetic.magnetic\"}],\"Right\":[{\"id\":\"S\",\"label\":\"S\",\"type\":\"foundation.magnetic.magnetic\"}],\"Top\":[]}"
  T8-T9 airgap : fl_lib/Magnetic/Magnetic Elements/Fundamental Reluctance  R=Rsl 1/H  phi_specify=off  phi_priority=None  phi=0 Wb  phi_nominal_specify=off  phi_nominal_value=1  phi_nominal_unit=Wb  mmf_specify=off  mmf_priority=None  mmf=0 A  mmf_nominal_specify=off  mmf_nominal_value=1  mmf_nominal_unit=A
      settings: InternalSimscapePortConfiguration="{\"Bottom\":[],\"Left\":[{\"id\":\"N\",\"label\":\"N\",\"type\":\"foundation.magnetic.magnetic\"}],\"Right\":[{\"id\":\"S\",\"label\":\"S\",\"type\":\"foundation.magnetic.magnetic\"}],\"Top\":[]}"
  T9-T1 airgap : fl_lib/Magnetic/Magnetic Elements/Fundamental Reluctance  R=Rsl 1/H  phi_specify=off  phi_priority=None  phi=0 Wb  phi_nominal_specify=off  phi_nominal_value=1  phi_nominal_unit=Wb  mmf_specify=off  mmf_priority=None  mmf=0 A  mmf_nominal_specify=off  mmf_nominal_value=1  mmf_nominal_unit=A
      settings: InternalSimscapePortConfiguration="{\"Bottom\":[],\"Left\":[{\"id\":\"N\",\"label\":\"N\",\"type\":\"foundation.magnetic.magnetic\"}],\"Right\":[{\"id\":\"S\",\"label\":\"S\",\"type\":\"foundation.magnetic.magnetic\"}],\"Top\":[]}"
  Tooth 1 (faulted) : ee_lib/Passive/Winding  Nw=Nws  Rw=Rw/3 Ohm  Rl=inf 1/H  Gw=gWinding 1/Ohm  thermalPort=simscape.enum.thermaleffects.omit  alpha=3.93e-3 1/K  Tmeas=25 degC  winding_thermal_mass=100 J/K  T_specify=off  T_priority=None  T=25 degC  T_nominal_specify=off  T_nominal_value=1  T_nominal_unit=degC  i_specify=off  i_priority=None  i=0 A  i_nominal_specify=off  i_nominal_value=1  i_nominal_unit=A  v_specify=off  v_priority=High  v=0 V  v_nominal_specify=off  v_nominal_value=1  v_nominal_unit=V  phi_specify=off  phi_priority=None  phi=0 Wb  phi_nominal_specify=off  phi_nominal_value=1  phi_nominal_unit=Wb  iterm_p_specify=off  iterm_p_priority=None  iterm_p=0 A  iterm_p_nominal_specify=off  iterm_p_nominal_value=1  iterm_p_nominal_unit=A  iterm_n_specify=off  iterm_n_priority=None  iterm_n=0 A  iterm_n_nominal_specify=off  iterm_n_nominal_value=1  iterm_n_nominal_unit=A  power_dissipated_specify=off  power_dissipated_priority=None  power_dissipated=0 W  power_dissipated_nominal_specify=off  power_dissipated_nominal_value=1  power_dissipated_nominal_unit=W
      settings: InternalSimscapePortConfiguration="{\"Bottom\":[],\"Left\":[{\"id\":\"p\",\"label\":\"+\",\"type\":\"foundation.electrical.electrical\"},{\"id\":\"n\",\"label\":\"-\",\"type\":\"foundation.electrical.electrical\"}],\"Right\":[{\"id\":\"N\",\"label\":\"N\",\"type\":\"foundation.magnetic.magnetic\"},{\"id\":\"S\",\"label\":\"S\",\"type\":\"foundation.magnetic.magnetic\"}],\"Top\":[]}"
  Tooth {2..9} (8 alike) : ee_lib/Passive/Winding  Nw=Nws  Rw=Rw/3 Ohm  Rl=inf 1/H  Gw=gWinding 1/Ohm  thermalPort=simscape.enum.thermaleffects.omit  alpha=3.93e-3 1/K  Tmeas=25 degC  winding_thermal_mass=100 J/K  T_specify=off  T_priority=None  T=25 degC  T_nominal_specify=off  T_nominal_value=1  T_nominal_unit=degC  i_specify=off  i_priority=None  i=0 A  i_nominal_specify=off  i_nominal_value=1  i_nominal_unit=A  v_specify=off  v_priority=None  v=0 V  v_nominal_specify=off  v_nominal_value=1  v_nominal_unit=V  phi_specify=off  phi_priority=None  phi=0 Wb  phi_nominal_specify=off  phi_nominal_value=1  phi_nominal_unit=Wb  iterm_p_specify=off  iterm_p_priority=None  iterm_p=0 A  iterm_p_nominal_specify=off  iterm_p_nominal_value=1  iterm_p_nominal_unit=A  iterm_n_specify=off  iterm_n_priority=None  iterm_n=0 A  iterm_n_nominal_specify=off  iterm_n_nominal_value=1  iterm_n_nominal_unit=A  power_dissipated_specify=off  power_dissipated_priority=None  power_dissipated=0 W  power_dissipated_nominal_specify=off  power_dissipated_nominal_value=1  power_dissipated_nominal_unit=W
      settings: InternalSimscapePortConfiguration="{\"Bottom\":[],\"Left\":[{\"id\":\"p\",\"label\":\"+\",\"type\":\"foundation.electrical.electrical\"},{\"id\":\"n\",\"label\":\"-\",\"type\":\"foundation.electrical.electrical\"}],\"Right\":[{\"id\":\"N\",\"label\":\"N\",\"type\":\"foundation.magnetic.magnetic\"},{\"id\":\"S\",\"label\":\"S\",\"type\":\"foundation.magnetic.magnetic\"}],\"Top\":[]}"
  tooth{1..9} (9 alike) : fl_lib/Magnetic/Magnetic Elements/Fundamental Reluctance  R=Rs 1/H  phi_specify=off  phi_priority=None  phi=0 Wb  phi_nominal_specify=off  phi_nominal_value=1  phi_nominal_unit=Wb  mmf_specify=off  mmf_priority=None  mmf=0 A  mmf_nominal_specify=off  mmf_nominal_value=1  mmf_nominal_unit=A
      settings: InternalSimscapePortConfiguration="{\"Bottom\":[],\"Left\":[{\"id\":\"N\",\"label\":\"N\",\"type\":\"foundation.magnetic.magnetic\"}],\"Right\":[{\"id\":\"S\",\"label\":\"S\",\"type\":\"foundation.magnetic.magnetic\"}],\"Top\":[]}"
  yoke{12,23,34,45,56,67,78,89,91} (9 alike) : fl_lib/Magnetic/Magnetic Elements/Fundamental Reluctance  R=Ry 1/H  phi_specify=off  phi_priority=None  phi=0 Wb  phi_nominal_specify=off  phi_nominal_value=1  phi_nominal_unit=Wb  mmf_specify=off  mmf_priority=None  mmf=0 A  mmf_nominal_specify=off  mmf_nominal_value=1  mmf_nominal_unit=A
      settings: InternalSimscapePortConfiguration="{\"Bottom\":[],\"Left\":[{\"id\":\"N\",\"label\":\"N\",\"type\":\"foundation.magnetic.magnetic\"}],\"Right\":[{\"id\":\"S\",\"label\":\"S\",\"type\":\"foundation.magnetic.magnetic\"}],\"Top\":[]}"
  A+ : PMIOPort  Side=Left
  B+ : PMIOPort  Port=2  Side=Left
  C+ : PMIOPort  Port=3  Side=Left
  A- : PMIOPort  Port=4  Side=Left
  B- : PMIOPort  Port=5  Side=Left
  C- : PMIOPort  Port=6  Side=Left
  R : PMIOPort  Port=7  Side=Right
  C : PMIOPort  Port=8  Side=Right
  connections:
  yoke91/RConn1 -- yoke12/LConn1 -- tooth1/LConn1
  Tooth 1 (faulted)/RConn2 -- Array Connection/LConn2 -- T2-T3 airgap/LConn1 -- T1-T2 airgap/RConn1
  T3-T4 airgap/LConn1 -- Array Connection/LConn3 -- Tooth 2/RConn2 -- T2-T3 airgap/RConn1
  Tooth 2/RConn1 -- tooth2/RConn1
  yoke91/LConn1 -- yoke89/RConn1 -- tooth9/LConn1
  yoke89/LConn1 -- Connection Label1/LConn1
  T9-T1 airgap/LConn1 -- Connection Label3/LConn1
  Tooth 9/LConn2 -- A+/RConn1
  Tooth 9/LConn1 -- Tooth 1 (faulted)/LConn1
  Tooth 1 (faulted)/LConn2 -- Tooth 2/LConn2
  Tooth 2/LConn1 -- A-/RConn1
  Tooth 9/RConn2 -- Array Connection/LConn1 -- T9-T1 airgap/RConn1 -- T1-T2 airgap/LConn1
  yoke45/LConn1 -- yoke34/RConn1 -- tooth4/LConn1
  Tooth 3/RConn2 -- Array Connection/LConn5 -- T5-T6 airgap/LConn1 -- T4-T5 airgap/RConn1
  T6-T7 airgap/LConn1 -- Array Connection/LConn6 -- T5-T6 airgap/RConn1 -- Tooth 4/RConn2
  yoke34/LConn1 -- yoke23/RConn1 -- tooth3/LConn1
  R/RConn1 -- Inertia/LConn1 -- Magnetic Rotor/LConn2
  Tooth 5/RConn2 -- Array Connection/LConn4 -- T3-T4 airgap/RConn1 -- T4-T5 airgap/LConn1
  yoke45/RConn1 -- yoke56/LConn1 -- tooth5/LConn1
  Tooth 5/LConn2 -- C+/RConn1
  Tooth 3/LConn2 -- Tooth 4/LConn2
  Tooth 5/LConn1 -- Tooth 3/LConn1
  Tooth 4/LConn1 -- C-/RConn1
  yoke78/LConn1 -- yoke67/RConn1 -- tooth7/LConn1
  Tooth 6/RConn2 -- Array Connection/LConn8 -- T8-T9 airgap/LConn1 -- T7-T8 airgap/RConn1
  T8-T9 airgap/RConn1 -- Array Connection/LConn9 -- Connection Label2/LConn1 -- Tooth 7/RConn2
  yoke67/LConn1 -- yoke56/RConn1 -- tooth6/LConn1
  Tooth 8/RConn2 -- Array Connection/LConn7 -- T6-T7 airgap/RConn1 -- T7-T8 airgap/LConn1
  C/RConn1 -- Magnetic Rotor/LConn1
  tooth8/LConn1 -- yoke78/RConn1 -- Connection Label/LConn1
  Tooth 8/LConn2 -- B+/RConn1
  Tooth 8/LConn1 -- Tooth 6/LConn1
  Tooth 6/LConn2 -- Tooth 7/LConn2
  Tooth 7/LConn1 -- B-/RConn1
  Tooth 1 (faulted)/RConn1 -- tooth1/RConn1
  yoke23/LConn1 -- tooth2/LConn1 -- yoke12/RConn1
  Tooth 5/RConn1 -- tooth3/RConn1
  Tooth 3/RConn1 -- tooth4/RConn1
  Tooth 4/RConn1 -- tooth5/RConn1
  Tooth 8/RConn1 -- tooth6/RConn1
  Tooth 6/RConn1 -- tooth7/RConn1
  Tooth 9/RConn1 -- tooth9/RConn1
  Tooth 7/RConn1 -- tooth8/RConn1
  Array Connection/RConn1 -- Magnetic Rotor/LConn3
  Array Connection1/RConn1 -- Magnetic Rotor/RConn1
  Array Connection1/LConn2 -- Array Connection1/LConn1 -- Array Connection1/LConn3 -- Array Connection1/LConn4 -- Magnetic Reference/LConn1 -- Array Connection1/LConn5 -- Array Connection1/LConn6 -- Array Connection1/LConn7 -- Array Connection1/LConn9 -- Array Connection1/LConn8

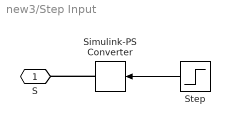
== system new3/Step Input ==
  Simulink-PS Converter : nesl_utility/Simulink-PS Converter  PhysicalDomain=network_engine_domain  SubClassName=ps_input  LeftPortType=input  RightPortType=output  PseudoPeriodic=off  Frequencies=[]  NoiseDistribution=none  NoiseParameters=[]  Unit=1  AffineConversion=off  FilteringAndDerivatives=zero  SimscapeFilterOrder=1  InputFilterTimeConstant=.001  UdotUserProvided=0
  Step : Step  Time=0.1  After=-0.24e-3  SampleTime=0
  S : PMIOPort  Side=Left
  wires:
  Step/1 -> Simulink-PS Converter/1
  connections:
  Simulink-PS Converter/RConn1 -- S/RConn1

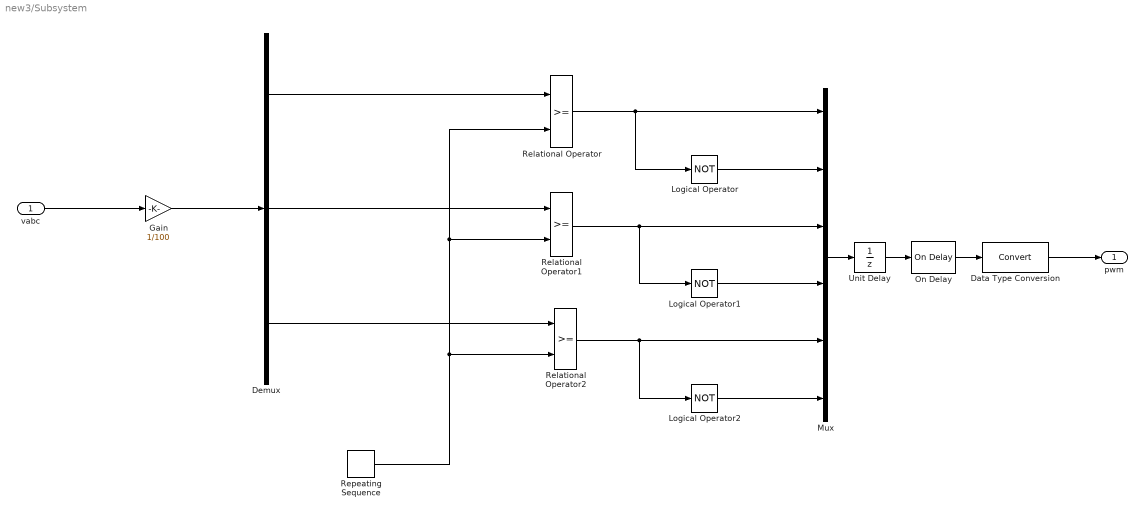
== system new3/Subsystem ==
  vabc : Inport
  Data Type Conversion : DataTypeConversion  SaturateOnIntegerOverflow=off  RndMeth=Floor
  Demux : Demux  Outputs=3
  Gain : Gain  Gain=1/100
  Logical Operator : Logic  Operator=NOT  AllPortsSameDT=off  OutDataTypeStr=boolean
  Logical Operator1 : Logic  Operator=NOT  AllPortsSameDT=off  OutDataTypeStr=boolean
  Logical Operator2 : Logic  Operator=NOT  AllPortsSameDT=off  OutDataTypeStr=boolean
  Mux : Mux  Inputs=6
  On Delay : spsOnDelayLib/On Delay  DelayType=On delay  delay=2e-6  ic=0  Ts=2e-6
  Relational Operator : RelationalOperator  OutDataTypeStr=boolean  RndMeth=Simplest  InputSameDT=off
  Relational Operator1 : RelationalOperator  OutDataTypeStr=boolean  RndMeth=Simplest  InputSameDT=off
  Relational Operator2 : RelationalOperator  OutDataTypeStr=boolean  RndMeth=Simplest  InputSameDT=off
  Repeating Sequence : simulink/Sources/Repeating Sequence  rep_seq_t=[0 0.0001]  rep_seq_y=[-1 1]
  Unit Delay : UnitDelay  SampleTime=-1  HasFrameUpgradeWarning=on
  pwm : Outport  VectorParamsAs1DForOutWhenUnconnected=off
  wires:
  Repeating Sequence/1 -> Relational Operator2/2, Relational Operator/2, Relational Operator1/2
  Demux/1 -> Relational Operator/1
  Relational Operator/1 -> Mux/1, Logical Operator/1
  Logical Operator/1 -> Mux/2
  Logical Operator1/1 -> Mux/4
  Demux/2 -> Relational Operator1/1
  Relational Operator1/1 -> Logical Operator1/1, Mux/3
  Logical Operator2/1 -> Mux/6
  Demux/3 -> Relational Operator2/1
  Relational Operator2/1 -> Logical Operator2/1, Mux/5
  Mux/1 -> Unit Delay/1
  vabc/1 -> Gain/1
  Gain/1 -> Demux/1
  Data Type Conversion/1 -> pwm/1
  Unit Delay/1 -> On Delay/1
  On Delay/1 -> Data Type Conversion/1

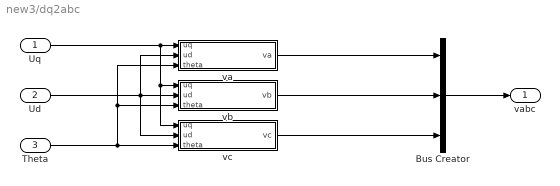
== system new3/dq2abc ==
  Uq : Inport
  Ud : Inport  Port=2
  Theta : Inport  Port=3
  Bus Creator : BusCreator  Inputs=3
  va : Subsystem
  vb : Subsystem
  vc : Subsystem
  vabc : Outport  VectorParamsAs1DForOutWhenUnconnected=off
  wires:
  vb/1(vb) -> Bus Creator/2
  Ud/1 -> va/2(ud), vb/2(ud), vc/2(ud)
  Uq/1 -> vc/1(uq), vb/1(uq), va/1(uq)
  va/1(va) -> Bus Creator/1
  Theta/1 -> va/3(theta), vb/3(theta), vc/3(theta)
  vc/1(vc) -> Bus Creator/3
  Bus Creator/1 -> vabc/1

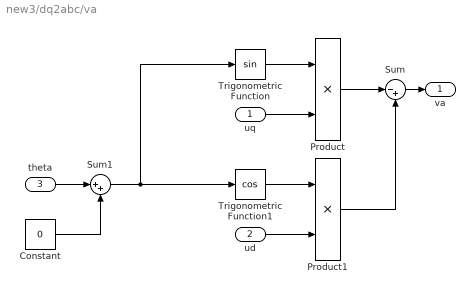
== system new3/dq2abc/va ==
  uq : Inport
  ud : Inport  Port=2
  theta : Inport  Port=3
  Constant : Constant  Value=0
  Product : Product
  Product1 : Product
  Sum : Sum  Inputs=|-+
  Sum1 : Sum  Inputs=|++
  Trigonometric Function : Trigonometry
  Trigonometric Function1 : Trigonometry  Operator=cos
  va : Outport  VectorParamsAs1DForOutWhenUnconnected=off
  wires:
  Product1/1 -> Sum/2
  Product/1 -> Sum/1
  ud/1 -> Product1/2
  Trigonometric Function/1 -> Product/1
  Trigonometric Function1/1 -> Product1/1
  Sum/1 -> va/1
  uq/1 -> Product/2
  Constant/1 -> Sum1/2
  theta/1 -> Sum1/1
  Sum1/1 -> Trigonometric Function1/1, Trigonometric Function/1

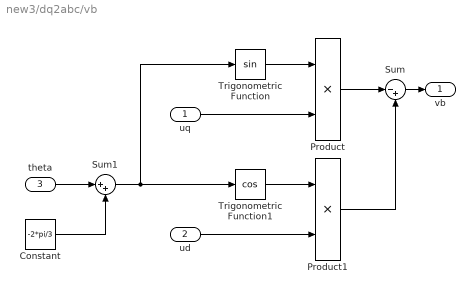
== system new3/dq2abc/vb ==
  uq : Inport
  ud : Inport  Port=2
  theta : Inport  Port=3
  Constant : Constant  Value=-2*pi/3
  Product : Product
  Product1 : Product
  Sum : Sum  Inputs=|-+
  Sum1 : Sum  Inputs=|++
  Trigonometric Function : Trigonometry
  Trigonometric Function1 : Trigonometry  Operator=cos
  vb : Outport  VectorParamsAs1DForOutWhenUnconnected=off
  wires:
  Product1/1 -> Sum/2
  Product/1 -> Sum/1
  ud/1 -> Product1/2
  Trigonometric Function/1 -> Product/1
  Trigonometric Function1/1 -> Product1/1
  Sum/1 -> vb/1
  uq/1 -> Product/2
  Constant/1 -> Sum1/2
  theta/1 -> Sum1/1
  Sum1/1 -> Trigonometric Function1/1, Trigonometric Function/1

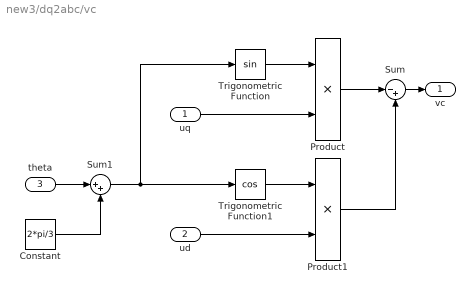
== system new3/dq2abc/vc ==
  uq : Inport
  ud : Inport  Port=2
  theta : Inport  Port=3
  Constant : Constant  Value=2*pi/3
  Product : Product
  Product1 : Product
  Sum : Sum  Inputs=|-+
  Sum1 : Sum  Inputs=|++
  Trigonometric Function : Trigonometry
  Trigonometric Function1 : Trigonometry  Operator=cos
  vc : Outport  VectorParamsAs1DForOutWhenUnconnected=off
  wires:
  Product1/1 -> Sum/2
  Product/1 -> Sum/1
  ud/1 -> Product1/2
  Trigonometric Function/1 -> Product/1
  Trigonometric Function1/1 -> Product1/1
  Sum/1 -> vc/1
  uq/1 -> Product/2
  Constant/1 -> Sum1/2
  theta/1 -> Sum1/1
  Sum1/1 -> Trigonometric Function1/1, Trigonometric Function/1
